simulink model "mvdc_curvvel_tracking"  (R2018b)
settings: configuration reference "Active" (kept outside this file)
undefined symbols (not defined in the file): A_VehicleReference_m2, drag_coefficient, l_front_m, l_rear_m, P_VDC_CurvDistActive, P_VDC_CurvDistEst_PT1_s, P_VDC_CurvKp, P_VDC_EmergencyBrakeAcceleration_mps2, P_VDC_EnterStandstillThreshhold_mps, P_VDC_FullControlSpeed_mps, P_VDC_FxMaxDistComp_N, P_VDC_FxMaxDistFF_N, P_VDC_FxMaxFB_N, P_VDC_FxMaxFF_N, P_VDC_FxMaxSlope_Nps, P_VDC_FxMinDistComp_N, P_VDC_FxMinDistFF_N, P_VDC_FxMinFB_N, P_VDC_FxMinFF_N, P_VDC_FxMinSlope_Nps, P_VDC_LatDeltaMaxDistComp_rad, P_VDC_LatDeltaMaxFB_rad, P_VDC_LatDeltaMaxFF_rad, P_VDC_LatDeltaMinDistComp_rad, P_VDC_LatDeltaMinFB_rad, P_VDC_LatDeltaMinFF_rad, P_VDC_LongKp, P_VDC_LowPassUSCT1, P_VDC_MaxSlopeDelta_radps, P_VDC_MinSlopeDelta_radps, P_VDC_NegativeFxStandstill_N, P_VDC_SlowControlSpeed_mps, P_VDC_UndersteerCompensationActive_b, P_VDC_UndersteerCompensationLowPassActive_b, P_VDC_UndersteerGradient, P_VDC_UseManualFF, P_VDC_VelCon_vMaxStatic_mps, P_VDC_VelDistEst_PT1_s, P_VDC_VelDistFBActive, P_VDC_VelDistFFActive, roh_air, tS, tyreradius_front_m, tyreradius_rear_m, vehiclemass_kg, WheelInertia_Front_kgm2, WheelInertia_Rear_kgm2
libraries: simulink x7, rr_general x7
settings Model: DataDictionary=mvdc_curvvel_tracking.sldd  Creator=wischnewski  LastModifiedBy=ge34qer

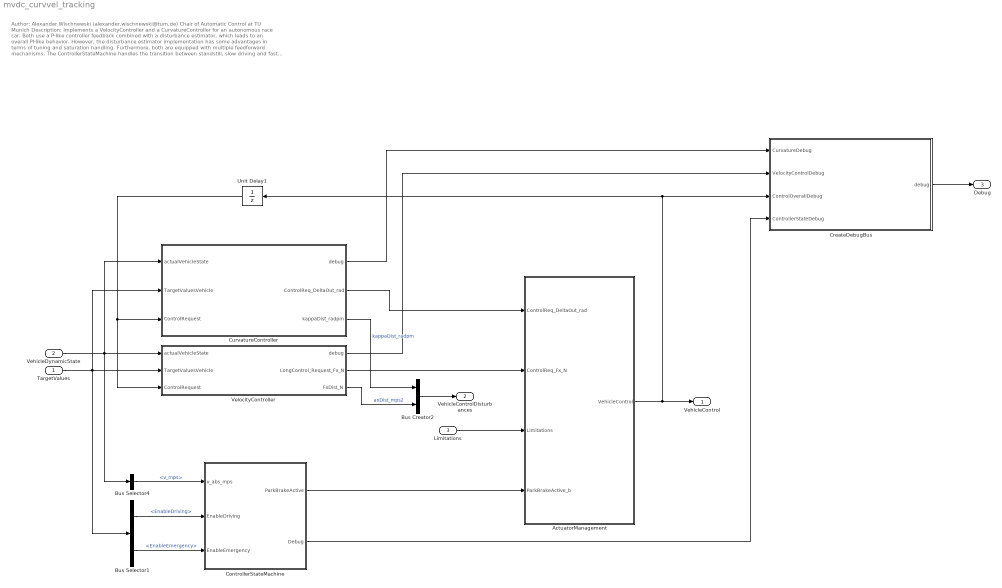
== system mvdc_curvvel_tracking ==
  note: Author: Alexander Wischnewski (alexander.wischnewski@tum.de)
      | Chair of Automatic Control at TU Munich
      |
      | Description: Implements a VelocityController and a CurvatureController for an autonomous race car. Both use a P-like controller feedback
      | combined with a disturbance estimator, which leads to an overall PI-like behavior. However, the disturbance estimator
      | implementation has some advantages in terms of tuning and saturation handling. Furthermore, both are equipped with multiple
      | feedforward mechanisms.
      |
      | The ControllerStateMachine handles the transition between standstill, slow driving and fast driving. This allows different
      | controller configurations in these scenarios.
      |
      | ActuatorManagement takes care of the final checks before the setpoints are passed to the low level actuators.
      |
      | Inputs:
      | TargetValues Setpoints and necessary feedforward information for both controllers
      | VehicleDynamicState Fused vehicle state (position, velocities, accelerations, etc.)
      | Limitations Actuator limitations
      |
      | Outputs:
      | VehicleControl Actuator setpoints used to control the vehicle
      | VehicleControlDisturbances Disturbance estimates to be used for diagnosis of vehicle status
      | Debug debug bus which includes all component debug information
  TargetValues : Inport  OutDataTypeStr=Bus: TargetValuesVehicleDynamics  PortDimensions=1  BusOutputAsStruct=on
  VehicleDynamicState : Inport  Port=2  OutDataTypeStr=Bus: VehicleDynamicState
  Limitations : Inport  Port=3  OutDataTypeStr=Bus: ActuatorLimitations  PortDimensions=1  BusOutputAsStruct=on
  ActuatorManagement : Subsystem
  Bus Creator2 : BusCreator  Inputs=2  OutDataTypeStr=Bus: VehicleControlDisturbances
      settings: InheritFromInputs=off
  Bus Selector1 : BusSelector  OutputSignals=EnableDriving,EnableEmergency
  Bus Selector4 : BusSelector  OutputSignals=v_mps
  ControllerStateMachine : Subsystem
  CreateDebugBus : Subsystem
  CurvatureController : Subsystem
  Unit Delay1 : UnitDelay  SampleTime=-1
  VelocityController : Subsystem
  VehicleControl : Outport  OutDataTypeStr=Bus: VehicleControl  BusOutputAsStruct=on
  VehicleControlDisturbances : Outport  Port=2  OutDataTypeStr=Bus: VehicleControlDisturbances  BusOutputAsStruct=on
  Debug : Outport  Port=3  OutDataTypeStr=Bus: mvdc_curvvel_tracking_debug  BusOutputAsStruct=on
  wires:
  ActuatorManagement/1(VehicleControl) -> VehicleControl/1, Unit Delay1/1, CreateDebugBus/3(ControlOverallDebug)
  VehicleDynamicState/1 -> CurvatureController/1(actualVehicleState), Bus Selector4/1, VelocityController/1(actualVehicleState)
  TargetValues/1 -> Bus Selector1/1, CurvatureController/2(TargetValuesVehicle), VelocityController/2(TargetValuesVehicle)
  Bus Selector4/1 -> ControllerStateMachine/1(v_abs_mps)  "<v_mps>"
  CurvatureController/2(ControlReq_DeltaOut_rad) -> ActuatorManagement/1(ControlReq_DeltaOut_rad)
  VelocityController/2(LongControl_Request_Fx_N) -> ActuatorManagement/2(ControlReq_Fx_N)
  Bus Creator2/1 -> VehicleControlDisturbances/1
  VelocityController/3(FxDist_N) -> Bus Creator2/2  "axDist_mps2"
  CurvatureController/3(kappaDist_radpm) -> Bus Creator2/1  "kappaDist_radpm"
  Limitations/1 -> ActuatorManagement/3(Limitations)
  Bus Selector1/1 -> ControllerStateMachine/2(EnableDriving)  "<EnableDriving>"
  Bus Selector1/2 -> ControllerStateMachine/3(EnableEmergency)  "<EnableEmergency>"
  Unit Delay1/1 -> CurvatureController/3(ControlRequest), VelocityController/3(ControlRequest)
  CurvatureController/1(debug) -> CreateDebugBus/1(CurvatureDebug)
  VelocityController/1(debug) -> CreateDebugBus/2(VelocityControlDebug)
  ControllerStateMachine/2(Debug) -> CreateDebugBus/4(ControllerStateDebug)
  CreateDebugBus/1(debug) -> Debug/1
  ControllerStateMachine/1("ParkBrakeActive ") -> ActuatorManagement/4(ParkBrakeActive_b)

== system mvdc_curvvel_tracking/ActuatorManagement ==
  ControlReq_DeltaOut_rad : Inport
  ControlReq_Fx_N : Inport  Port=2
  Limitations : Inport  Port=3
  ParkBrakeActive_b : Inport  Port=4
  Bus Creator : BusCreator  Inputs=3  OutDataTypeStr=Bus: VehicleControl
      settings: InheritFromInputs=off
  OutputChecksLong : Subsystem
  OutputChecksSteering : Subsystem
  VehicleControl : Outport  OutDataTypeStr=Bus: VehicleControl  BusOutputAsStruct=on
  wires:
  Limitations/1 -> OutputChecksLong/1(Limitations), OutputChecksSteering/1(Limitations)
  ParkBrakeActive_b/1 -> Bus Creator/3  "ParkBrakeActive"
  Bus Creator/1 -> VehicleControl/1
  ControlReq_DeltaOut_rad/1 -> OutputChecksSteering/2(delta_SteeringAngleRequest_radpm)
  OutputChecksSteering/1(RequestSteeringAngle_rad) -> Bus Creator/1  "RequestSteeringAngle_rad"
  ControlReq_Fx_N/1 -> OutputChecksLong/2(Fx_LongControlRequest_N)
  OutputChecksLong/1(RequestLongForce_N) -> Bus Creator/2  "RequestLongForce_N"

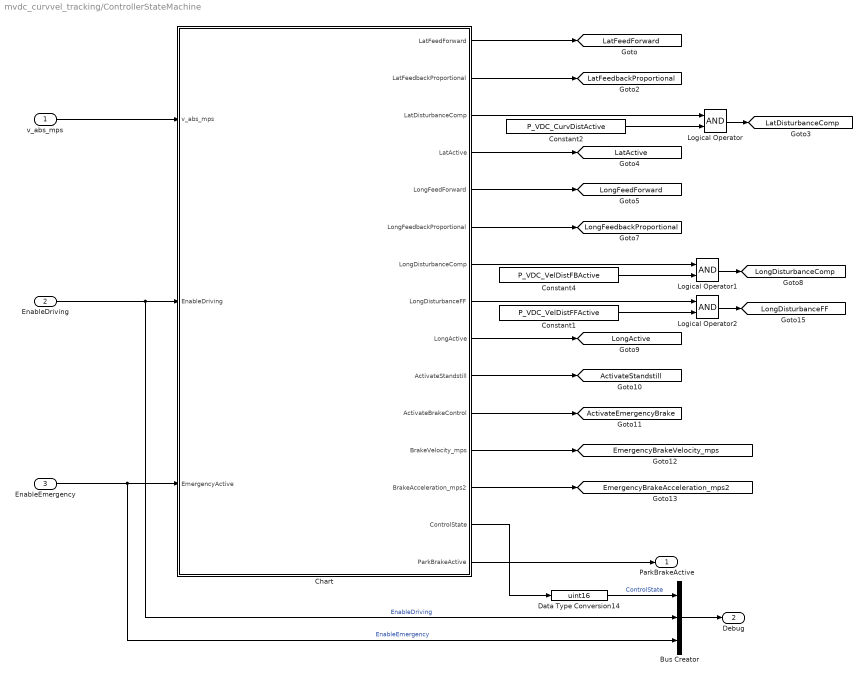
== system mvdc_curvvel_tracking/ControllerStateMachine ==
  v_abs_mps : Inport
  EnableDriving : Inport  Port=2
  EnableEmergency : Inport  Port=3
  Bus Creator : BusCreator  Inputs=3
  Chart : Stateflow chart  TreatAsAtomicUnit=on
  Constant1 : Constant  Value=P_VDC_VelDistFFActive
  Constant2 : Constant  Value=P_VDC_CurvDistActive
  Constant4 : Constant  Value=P_VDC_VelDistFBActive
  Data Type Conversion14 : DataTypeConversion  OutDataTypeStr=uint16
  Logical Operator : Logic  AllPortsSameDT=off  OutDataTypeStr=boolean
  Logical Operator1 : Logic  AllPortsSameDT=off  OutDataTypeStr=boolean
  Logical Operator2 : Logic  AllPortsSameDT=off  OutDataTypeStr=boolean
  "ParkBrakeActive " : Outport  BusOutputAsStruct=on
  Debug : Outport  Port=2
  tag scope: ActivateEmergencyBrake=global, ActivateStandstill=global, EmergencyBrakeAcceleration_mps2=global, EmergencyBrakeVelocity_mps=global, LatActive=global, LatDisturbanceComp=global, LatFeedForward=global, LatFeedbackProportional=global, LongActive=global, LongDisturbanceComp=global, LongDisturbanceFF=global, LongFeedForward=global, LongFeedbackProportional=global
  wires:
  Chart/2(LatFeedbackProportional) -> [LatFeedbackProportional]
  Chart/1(LatFeedForward) -> [LatFeedForward]
  Chart/9(LongActive) -> [LongActive]
  Logical Operator/1 -> [LatDisturbanceComp]
  Constant2/1 -> Logical Operator/2
  Constant4/1 -> Logical Operator1/2
  Logical Operator1/1 -> [LongDisturbanceComp]
  Chart/11(ActivateBrakeControl) -> [ActivateEmergencyBrake]
  Chart/13(BrakeAcceleration_mps2) -> [EmergencyBrakeAcceleration_mps2]
  Chart/12(BrakeVelocity_mps) -> [EmergencyBrakeVelocity_mps]
  Chart/10(ActivateStandstill) -> [ActivateStandstill]
  v_abs_mps/1 -> Chart/1(v_abs_mps)
  Chart/7(LongDisturbanceComp) -> Logical Operator1/1
  Chart/4(LatActive) -> [LatActive]
  Chart/5(LongFeedForward) -> [LongFeedForward]
  Chart/6(LongFeedbackProportional) -> [LongFeedbackProportional]
  Chart/3(LatDisturbanceComp) -> Logical Operator/1
  Constant1/1 -> Logical Operator2/2
  Logical Operator2/1 -> [LongDisturbanceFF]
  Chart/8(LongDisturbanceFF) -> Logical Operator2/1
  EnableDriving/1 -> Bus Creator/2, Chart/2(EnableDriving)  "EnableDriving"
  EnableEmergency/1 -> Bus Creator/3, Chart/3(EmergencyActive)  "EnableEmergency"
  Bus Creator/1 -> Debug/1
  Chart/14(ControlState) -> Data Type Conversion14/1
  Data Type Conversion14/1 -> Bus Creator/1  "ControlState"
  Chart/15(ParkBrakeActive) -> "ParkBrakeActive "/1

== system mvdc_curvvel_tracking/CreateDebugBus ==
  CurvatureDebug : Inport
  VelocityControlDebug : Inport  Port=2
  ControlOverallDebug : Inport  Port=3
  ControllerStateDebug : Inport  Port=4
  Bus Creator1 : BusCreator  Inputs=17
  Bus Selector : BusSelector  OutputSignals=Long_FB_Dist_FxReq_N,Long_FF_Dist_FxReq_N,Long_FB_VelDiff_FxReq_N,Long_FF_Traj_FxReq_N,Long_VelError_mps,Long_TargetSpeed_mps,Long_axTarget_mps2
  Bus Selector2 : BusSelector  OutputSignals=Curv_all_KappaReq_radpm,Curv_FB_Dist_DeltaReq_rad,Curv_FB_Diff_DeltaReq_rad,Curv_FF_Kappa_DeltaReq_rad,Curv_CurvError_radpm,Curv_TargetCurv_radpm
  Bus Selector3 : BusSelector  OutputSignals=ControlState,EnableDriving,EnableEmergency
  debug : Outport
  wires:
  Bus Selector/3 -> Bus Creator1/9  "<Long_FB_VelDiff_FxReq_N>"
  Bus Selector/4 -> Bus Creator1/10  "<Long_FF_Traj_FxReq_N>"
  Bus Selector/1 -> Bus Creator1/7  "<Long_FB_Dist_FxReq_N>"
  Bus Selector/5 -> Bus Creator1/11  "<Long_VelError_mps>"
  Bus Selector2/6 -> Bus Creator1/6  "<Curv_TargetCurv_radpm>"
  Bus Selector2/4 -> Bus Creator1/4  "<Curv_FF_Kappa_DeltaReq_rad>"
  Bus Selector3/2 -> Bus Creator1/16  "<EnableDriving>"
  VelocityControlDebug/1 -> Bus Selector/1
  Bus Selector2/3 -> Bus Creator1/3  "<Curv_FB_Diff_DeltaReq_rad>"
  Bus Selector3/1 -> Bus Creator1/15  "<ControlState>"
  ControllerStateDebug/1 -> Bus Selector3/1
  Bus Selector2/1 -> Bus Creator1/1  "<Curv_all_KappaReq_radpm>"
  Bus Selector2/5 -> Bus Creator1/5  "<Curv_CurvError_radpm>"
  Bus Selector3/3 -> Bus Creator1/17  "<EnableEmergency>"
  Bus Selector2/2 -> Bus Creator1/2  "<Curv_FB_Dist_DeltaReq_rad>"
  Bus Creator1/1 -> debug/1
  ControlOverallDebug/1 -> Bus Creator1/14  "CO"
  Bus Selector/7 -> Bus Creator1/13  "<Long_axTarget_mps2>"
  Bus Selector/2 -> Bus Creator1/8  "<Long_FF_Dist_FxReq_N>"
  CurvatureDebug/1 -> Bus Selector2/1
  Bus Selector/6 -> Bus Creator1/12  "<Long_TargetSpeed_mps>"

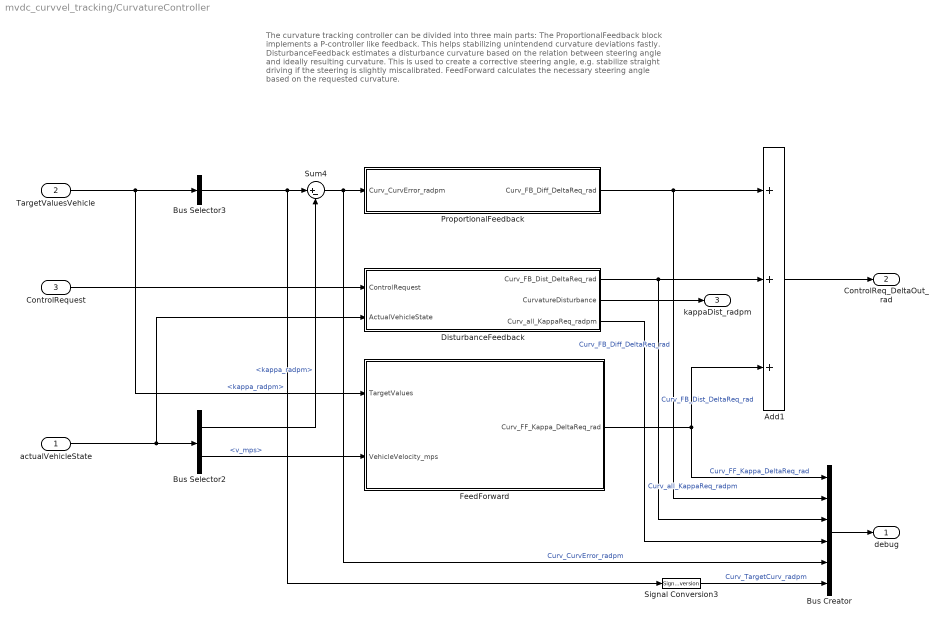
== system mvdc_curvvel_tracking/CurvatureController ==
  note: The curvature tracking controller can be divided into three main parts:
      |
      | The ProportionalFeedback block implements a P-controller like feedback. This helps stabilizing unintendend curvature deviations fastly.
      |
      | DisturbanceFeedback estimates a disturbance curvature based on the relation between steering angle and ideally resulting curvature. This is
      | used to create a corrective steering angle, e.g. stabilize straight driving if the steering is slightly miscalibrated.
      |
      | FeedForward calculates the necessary steering angle based on the requested curvature.
  actualVehicleState : Inport
  TargetValuesVehicle : Inport  Port=2
  ControlRequest : Inport  Port=3
  Add1 : Sum  Inputs=+++
  Bus Creator : BusCreator  Inputs=6
  Bus Selector2 : BusSelector  OutputSignals=kappa_radpm,v_mps
  Bus Selector3 : BusSelector  OutputSignals=kappa_radpm
  DisturbanceFeedback : Subsystem
  FeedForward : Subsystem
  ProportionalFeedback : Subsystem
  Signal Conversion3 : SignalConversion  OverrideOpt=off
  Sum4 : Sum  Inputs=|+-
  debug : Outport
  ControlReq_DeltaOut_rad : Outport  Port=2
  kappaDist_radpm : Outport  Port=3
  wires:
  Bus Selector2/1 -> Sum4/2  "<kappa_radpm>"
  Sum4/1 -> Bus Creator/5, ProportionalFeedback/1(Curv_CurvError_radpm)  "Curv_CurvError_radpm"
  Bus Selector2/2 -> FeedForward/2(VehicleVelocity_mps)  "<v_mps>"
  actualVehicleState/1 -> DisturbanceFeedback/2(ActualVehicleState), Bus Selector2/1
  TargetValuesVehicle/1 -> FeedForward/1(TargetValues), Bus Selector3/1
  Signal Conversion3/1 -> Bus Creator/6  "Curv_TargetCurv_radpm"
  Bus Creator/1 -> debug/1
  Bus Selector3/1 -> Sum4/1, Signal Conversion3/1  "<kappa_radpm>"
  Add1/1 -> ControlReq_DeltaOut_rad/1
  ProportionalFeedback/1(Curv_FB_Diff_DeltaReq_rad) -> Add1/1, Bus Creator/2  "Curv_FB_Diff_DeltaReq_rad"
  DisturbanceFeedback/1(Curv_FB_Dist_DeltaReq_rad) -> Add1/2, Bus Creator/3  "Curv_FB_Dist_DeltaReq_rad"
  FeedForward/1(Curv_FF_Kappa_DeltaReq_rad) -> Bus Creator/1, Add1/3  "Curv_FF_Kappa_DeltaReq_rad"
  ControlRequest/1 -> DisturbanceFeedback/1(ControlRequest)
  DisturbanceFeedback/2(CurvatureDisturbance) -> kappaDist_radpm/1
  DisturbanceFeedback/3(Curv_all_KappaReq_radpm) -> Bus Creator/4  "Curv_all_KappaReq_radpm"

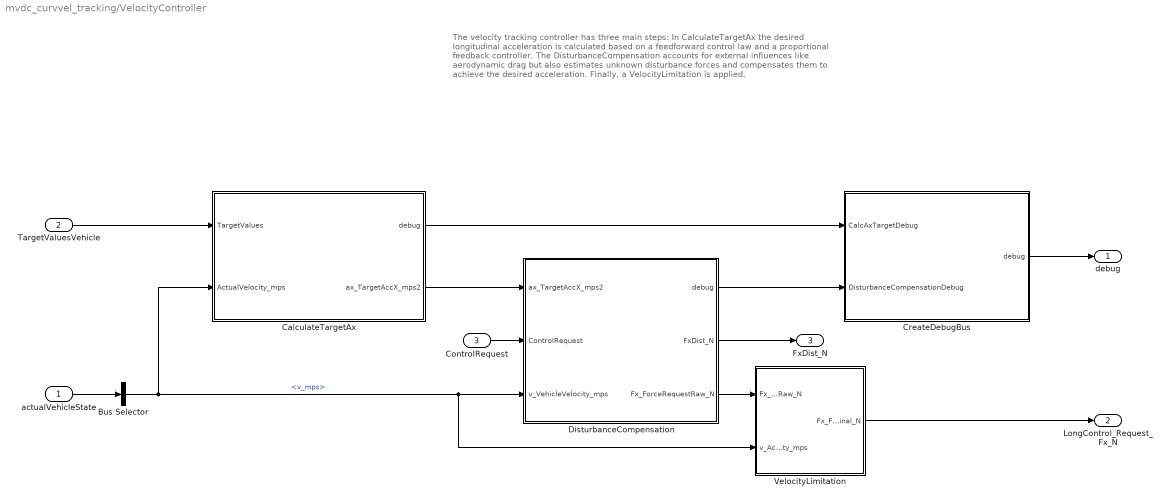
== system mvdc_curvvel_tracking/VelocityController ==
  note: The velocity tracking controller has three main steps:
      |
      | In CalculateTargetAx the desired longitudinal acceleration is calculated based on a
      | feedforward control law and a proportional feedback controller.
      |
      | The DisturbanceCompensation accounts for external influences like aerodynamic drag
      | but also estimates unknown disturbance forces and compensates them to achieve
      | the desired acceleration.
      |
      | Finally, a VelocityLimitation is applied.
  actualVehicleState : Inport
  TargetValuesVehicle : Inport  Port=2
  ControlRequest : Inport  Port=3
  Bus Selector : BusSelector  OutputSignals=v_mps
  CalculateTargetAx : Subsystem
  CreateDebugBus : Subsystem
  DisturbanceCompensation : Subsystem
  VelocityLimitation : Subsystem
  debug : Outport
  LongControl_Request_Fx_N : Outport  Port=2
  FxDist_N : Outport  Port=3
  wires:
  Bus Selector/1 -> VelocityLimitation/2(v_ActualVelocity_mps), DisturbanceCompensation/3(v_VehicleVelocity_mps), CalculateTargetAx/2(ActualVelocity_mps)  "<v_mps>"
  TargetValuesVehicle/1 -> CalculateTargetAx/1(TargetValues)
  actualVehicleState/1 -> Bus Selector/1
  DisturbanceCompensation/2(FxDist_N) -> FxDist_N/1
  VelocityLimitation/1(Fx_ForceRequestFinal_N) -> LongControl_Request_Fx_N/1
  CalculateTargetAx/2(ax_TargetAccX_mps2) -> DisturbanceCompensation/1(ax_TargetAccX_mps2)
  ControlRequest/1 -> DisturbanceCompensation/2(ControlRequest)
  DisturbanceCompensation/3(Fx_ForceRequestRaw_N) -> VelocityLimitation/1(Fx_ForceRequestRaw_N)
  CalculateTargetAx/1(debug) -> CreateDebugBus/1(CalcAxTargetDebug)
  DisturbanceCompensation/1(debug) -> CreateDebugBus/2(DisturbanceCompensationDebug)
  CreateDebugBus/1(debug) -> debug/1

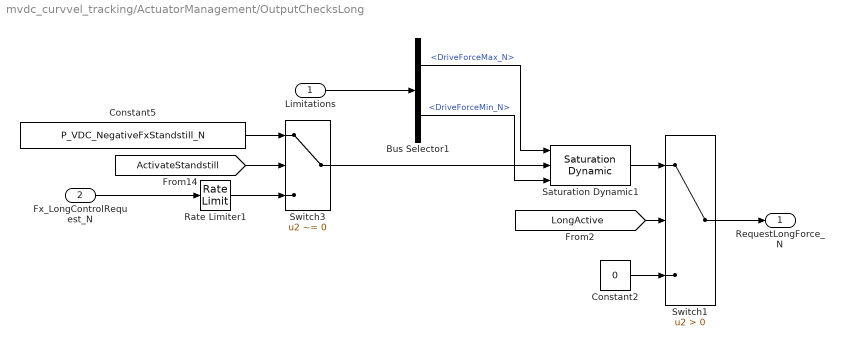
== system mvdc_curvvel_tracking/ActuatorManagement/OutputChecksLong ==
  Limitations : Inport
  Fx_LongControlRequest_N : Inport  Port=2
  Bus Selector1 : BusSelector  OutputSignals=DriveForceMax_N,DriveForceMin_N
  Constant2 : Constant  Value=0
  Constant5 : Constant  Value=P_VDC_NegativeFxStandstill_N
  Rate Limiter1 : RateLimiter  RisingSlewLimit=P_VDC_FxMaxSlope_Nps  FallingSlewLimit=P_VDC_FxMinSlope_Nps  SampleTimeMode=inherited
  Saturation Dynamic1 : simulink/Discontinuities/Saturation Dynamic  OutMin=[]  OutMax=[]  OutDataTypeStr=Inherit: Same as second input  OutDataType=fixdt(1, 16)  OutScaling=2^-10  DoSatur=off
  Switch1 : Switch  Criteria=u2 > Threshold
  Switch3 : Switch  Criteria=u2 ~= 0
  RequestLongForce_N : Outport
  wires:
  Saturation Dynamic1/1 -> Switch1/1
  Rate Limiter1/1 -> Switch3/3
  Bus Selector1/1 -> Saturation Dynamic1/1  "<DriveForceMax_N>"
  [ActivateStandstill] -> Switch3/2
  Constant2/1 -> Switch1/3
  Bus Selector1/2 -> Saturation Dynamic1/3  "<DriveForceMin_N>"
  Switch3/1 -> Saturation Dynamic1/2
  Constant5/1 -> Switch3/1
  [LongActive] -> Switch1/2
  Switch1/1 -> RequestLongForce_N/1
  Fx_LongControlRequest_N/1 -> Rate Limiter1/1
  Limitations/1 -> Bus Selector1/1

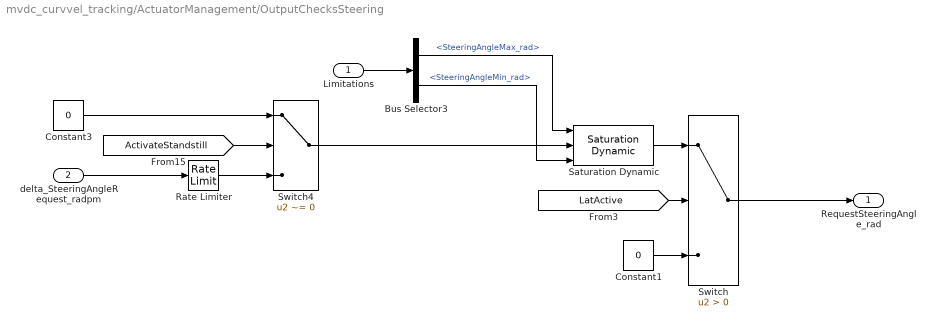
== system mvdc_curvvel_tracking/ActuatorManagement/OutputChecksSteering ==
  Limitations : Inport
  delta_SteeringAngleRequest_radpm : Inport  Port=2
  Bus Selector3 : BusSelector  OutputSignals=SteeringAngleMax_rad,SteeringAngleMin_rad
  Constant1 : Constant  Value=0
  Constant3 : Constant  Value=0
  Rate Limiter : RateLimiter  RisingSlewLimit=P_VDC_MaxSlopeDelta_radps  FallingSlewLimit=P_VDC_MinSlopeDelta_radps  SampleTimeMode=inherited
  Saturation Dynamic : simulink/Discontinuities/Saturation Dynamic  OutMin=[]  OutMax=[]  OutDataTypeStr=Inherit: Same as second input  OutDataType=fixdt(1, 16)  OutScaling=2^-10  DoSatur=off
  Switch : Switch  Criteria=u2 > Threshold
  Switch4 : Switch  Criteria=u2 ~= 0
  RequestSteeringAngle_rad : Outport
  wires:
  Switch4/1 -> Saturation Dynamic/2
  Constant3/1 -> Switch4/1
  Saturation Dynamic/1 -> Switch/1
  [ActivateStandstill] -> Switch4/2
  Rate Limiter/1 -> Switch4/3
  Bus Selector3/1 -> Saturation Dynamic/1  "<SteeringAngleMax_rad>"
  Bus Selector3/2 -> Saturation Dynamic/3  "<SteeringAngleMin_rad>"
  Constant1/1 -> Switch/3
  [LatActive] -> Switch/2
  delta_SteeringAngleRequest_radpm/1 -> Rate Limiter/1
  Switch/1 -> RequestSteeringAngle_rad/1
  Limitations/1 -> Bus Selector3/1

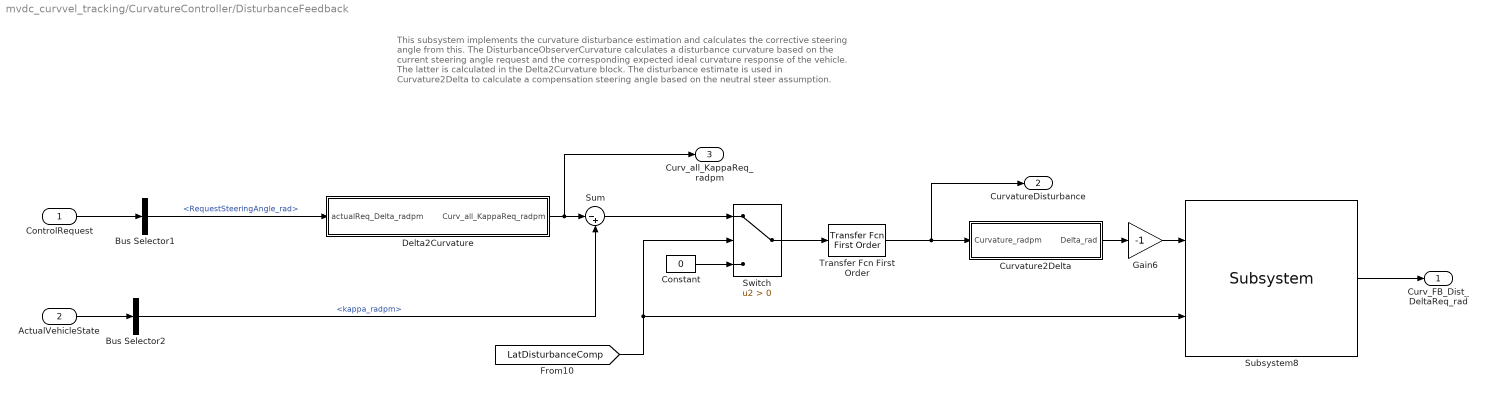
== system mvdc_curvvel_tracking/CurvatureController/DisturbanceFeedback ==
  note: This subsystem implements the curvature disturbance estimation and calculates the corrective steering angle from this.
      |
      | The DisturbanceObserverCurvature calculates a disturbance curvature based on the current steering angle request
      | and the corresponding expected ideal curvature response of the vehicle. The latter is calculated in the Delta2Curvature block.
      | The disturbance estimate is used in Curvature2Delta to calculate a compensation steering angle based on the neutral
      | steer assumption.
  ControlRequest : Inport
  ActualVehicleState : Inport  Port=2
  Bus Selector1 : BusSelector  OutputSignals=RequestSteeringAngle_rad
  Bus Selector2 : BusSelector  OutputSignals=kappa_radpm
  Constant : Constant  Value=0
  Curvature2Delta : Subsystem
  Delta2Curvature : Subsystem
  Gain6 : Gain  Gain=-1
  Subsystem8 : rr_general/Subsystem  UpperLimit=P_VDC_LatDeltaMaxDistComp_rad  LowerLimit=P_VDC_LatDeltaMinDistComp_rad
  Sum : Sum  Inputs=|-+
  Switch : Switch  Criteria=u2 > Threshold
  Transfer Fcn First Order : simulink/Discrete/Transfer Fcn First Order  PoleZ=exp(-tS/P_VDC_CurvDistEst_PT1_s)  ICPrevOutput=0.0  DoSatur=off
      settings: SourceProductName=Simulink
  Curv_FB_Dist_DeltaReq_rad : Outport
  CurvatureDisturbance : Outport  Port=2
  Curv_all_KappaReq_radpm : Outport  Port=3
  wires:
  Gain6/1 -> Subsystem8/1
  [LatDisturbanceComp] -> Subsystem8/2, Switch/2
  Curvature2Delta/1(Delta_rad) -> Gain6/1
  Subsystem8/1 -> Curv_FB_Dist_DeltaReq_rad/1
  ControlRequest/1 -> Bus Selector1/1
  Delta2Curvature/1(Curv_all_KappaReq_radpm) -> Curv_all_KappaReq_radpm/1, Sum/1
  Transfer Fcn First Order/1 -> CurvatureDisturbance/1, Curvature2Delta/1(Curvature_radpm)
  ActualVehicleState/1 -> Bus Selector2/1
  Bus Selector2/1 -> Sum/2  "<kappa_radpm>"
  Sum/1 -> Switch/1
  Constant/1 -> Switch/3
  Switch/1 -> Transfer Fcn First Order/1
  Bus Selector1/1 -> Delta2Curvature/1(actualReq_Delta_radpm)  "<RequestSteeringAngle_rad>"

== system mvdc_curvvel_tracking/CurvatureController/FeedForward ==
  note: Two options are available for feedforward generation:
      |
      | The top option uses a direct feed-through of a externally
      | supplied steering angle.
      |
      | The bottom option calculates the steering feedforward based on the
      | curvature setpoint and an additional feedforward curvature value kappaFF_radpm.
  TargetValues : Inport
  VehicleVelocity_mps : Inport  Port=2
  Bus Selector : BusSelector  OutputSignals=ManualFF_Delta_rad,kappa_radpm,kappaFF_radpm
  Constant2 : Constant  Value=P_VDC_UseManualFF
  Curvature2Delta : Subsystem
  Subsystem7 : rr_general/Subsystem  UpperLimit=P_VDC_LatDeltaMaxFF_rad  LowerLimit=P_VDC_LatDeltaMinFF_rad
  Sum : Sum  Inputs=++|
  Switch3 : Switch  Criteria=u2 ~= 0
  Curv_FF_Kappa_DeltaReq_rad : Outport
  wires:
  [LatFeedForward] -> Subsystem7/2
  Constant2/1 -> Switch3/2
  Sum/1 -> Curvature2Delta/1(TargetCurvature_radpm)
  Switch3/1 -> Subsystem7/1
  Curvature2Delta/1(SteeringAngle_rad) -> Switch3/3
  Subsystem7/1 -> Curv_FF_Kappa_DeltaReq_rad/1
  TargetValues/1 -> Bus Selector/1
  Bus Selector/1 -> Switch3/1  "<ManualFF_Delta_rad>"
  VehicleVelocity_mps/1 -> Curvature2Delta/2(ActualVelocity_mps)
  Bus Selector/3 -> Sum/2  "<kappaFF_radpm>"
  Bus Selector/2 -> Sum/1  "<kappa_radpm>"

== system mvdc_curvvel_tracking/CurvatureController/ProportionalFeedback ==
  Curv_CurvError_radpm : Inport
  Gain3 : Gain  Gain=P_VDC_CurvKp
  Subsystem9 : rr_general/Subsystem  UpperLimit=P_VDC_LatDeltaMaxFB_rad  LowerLimit=P_VDC_LatDeltaMinFB_rad
  Curv_FB_Diff_DeltaReq_rad : Outport
  wires:
  [LatFeedbackProportional] -> Subsystem9/2
  Subsystem9/1 -> Curv_FB_Diff_DeltaReq_rad/1
  Curv_CurvError_radpm/1 -> Gain3/1
  Gain3/1 -> Subsystem9/1

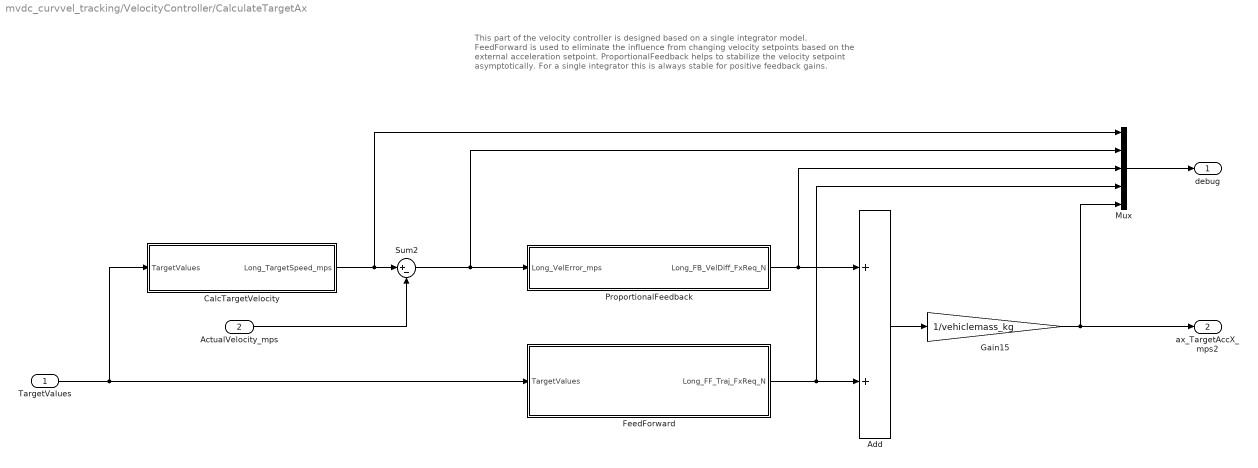
== system mvdc_curvvel_tracking/VelocityController/CalculateTargetAx ==
  note: This part of the velocity controller is designed based on a single integrator model.
      |
      | FeedForward is used to eliminate the influence from changing velocity setpoints based
      | on the external acceleration setpoint.
      |
      | ProportionalFeedback helps to stabilize the velocity setpoint asymptotically. For a single
      | integrator this is always stable for positive feedback gains.
  TargetValues : Inport
  ActualVelocity_mps : Inport  Port=2
  Add : Sum
  CalcTargetVelocity : Subsystem
  FeedForward : Subsystem
  Gain15 : Gain  Gain=1/vehiclemass_kg
  Mux : Mux  Inputs=5
  ProportionalFeedback : Subsystem
  Sum2 : Sum  Inputs=|+-
  debug : Outport
  ax_TargetAccX_mps2 : Outport  Port=2
  wires:
  TargetValues/1 -> CalcTargetVelocity/1(TargetValues), FeedForward/1(TargetValues)
  ProportionalFeedback/1(Long_FB_VelDiff_FxReq_N) -> Mux/3, Add/1
  FeedForward/1(Long_FF_Traj_FxReq_N) -> Mux/4, Add/2
  Add/1 -> Gain15/1
  Gain15/1 -> Mux/5, ax_TargetAccX_mps2/1
  Mux/1 -> debug/1
  CalcTargetVelocity/1(Long_TargetSpeed_mps) -> Mux/1, Sum2/1
  ActualVelocity_mps/1 -> Sum2/2
  Sum2/1 -> Mux/2, ProportionalFeedback/1(Long_VelError_mps)

== system mvdc_curvvel_tracking/VelocityController/CreateDebugBus ==
  CalcAxTargetDebug : Inport
  DisturbanceCompensationDebug : Inport  Port=2
  Bus Creator : BusCreator  Inputs=7
  Demux : Demux  Outputs=5
  Demux1 : Demux  Outputs=2
  debug : Outport
  wires:
  CalcAxTargetDebug/1 -> Demux/1
  Bus Creator/1 -> debug/1
  Demux/3 -> Bus Creator/3  "Long_FB_VelDiff_FxReq_N"
  Demux1/1 -> Bus Creator/6  "Long_FB_Dist_FxReq_N"
  Demux/1 -> Bus Creator/1  "Long_TargetSpeed_mps"
  Demux/2 -> Bus Creator/2  "Long_VelError_mps"
  Demux/4 -> Bus Creator/4  "Long_FF_Traj_FxReq_N"
  Demux/5 -> Bus Creator/5  "Long_axTarget_mps2"
  Demux1/2 -> Bus Creator/7  "Long_FF_Dist_FxReq_N"
  DisturbanceCompensationDebug/1 -> Demux1/1

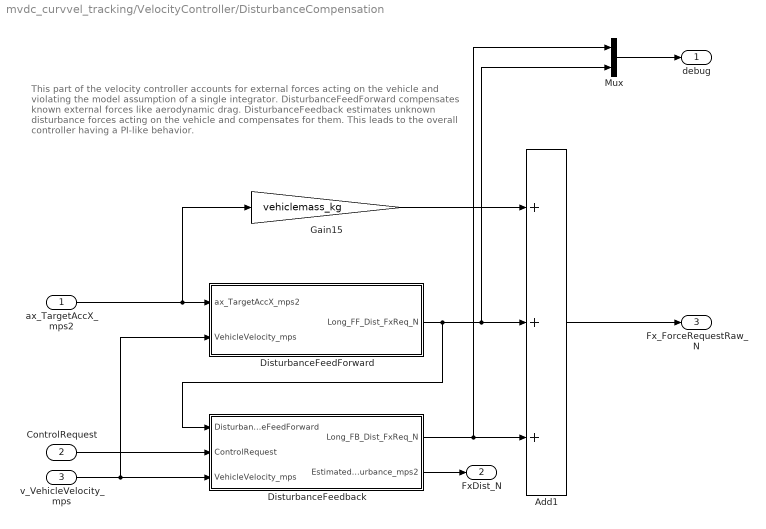
== system mvdc_curvvel_tracking/VelocityController/DisturbanceCompensation ==
  note: This part of the velocity controller accounts for external forces acting on the vehicle and
      | violating the model assumption of a single integrator.
      |
      | DisturbanceFeedForward compensates known external forces like aerodynamic drag.
      |
      | DisturbanceFeedback estimates unknown disturbance forces acting on the vehicle
      | and compensates for them. This leads to the overall controller having a PI-like behavior.
  ax_TargetAccX_mps2 : Inport
  ControlRequest : Inport  Port=2
  v_VehicleVelocity_mps : Inport  Port=3
  Add1 : Sum  Inputs=+++
  DisturbanceFeedForward : Subsystem
  DisturbanceFeedback : Subsystem
  Gain15 : Gain  Gain=vehiclemass_kg
  Mux : Mux  Inputs=2
  debug : Outport
  FxDist_N : Outport  Port=2
  Fx_ForceRequestRaw_N : Outport  Port=3
  wires:
  v_VehicleVelocity_mps/1 -> DisturbanceFeedForward/2(VehicleVelocity_mps), DisturbanceFeedback/3(VehicleVelocity_mps)
  DisturbanceFeedForward/1(Long_FF_Dist_FxReq_N) -> DisturbanceFeedback/1(DisturbanceFeedForward), Mux/2, Add1/2
  ControlRequest/1 -> DisturbanceFeedback/2(ControlRequest)
  Add1/1 -> Fx_ForceRequestRaw_N/1
  DisturbanceFeedback/1(Long_FB_Dist_FxReq_N) -> Mux/1, Add1/3
  ax_TargetAccX_mps2/1 -> Gain15/1, DisturbanceFeedForward/1(ax_TargetAccX_mps2)
  Gain15/1 -> Add1/1
  Mux/1 -> debug/1
  DisturbanceFeedback/2(EstimatedAccXDisturbance_mps2) -> FxDist_N/1

== system mvdc_curvvel_tracking/VelocityController/VelocityLimitation ==
  note: This subsystem implements a velocity limitation. If the vehicle reaches the velocity limit,
      | positive forces are no longer passed to the actuators.
  Fx_ForceRequestRaw_N : Inport
  v_ActualVelocity_mps : Inport  Port=2
  Compare To Zero : simulink/Logic and Bit Operations/Compare To Zero  relop=>=  OutDataTypeStr=boolean
  Constant1 : Constant  Value=P_VDC_VelCon_vMaxStatic_mps
  Saturation : Saturate  UpperLimit=0  LowerLimit=-inf
  Sum3 : Sum  Inputs=-+|
  Switch1 : Switch  Criteria=u2 > Threshold
  Fx_ForceRequestFinal_N : Outport
  wires:
  Fx_ForceRequestRaw_N/1 -> Switch1/3, Saturation/1
  Compare To Zero/1 -> Switch1/2
  Saturation/1 -> Switch1/1
  Switch1/1 -> Fx_ForceRequestFinal_N/1
  Sum3/1 -> Compare To Zero/1
  v_ActualVelocity_mps/1 -> Sum3/2
  Constant1/1 -> Sum3/1

== system mvdc_curvvel_tracking/CurvatureController/DisturbanceFeedback/Curvature2Delta ==
  Curvature_radpm : Inport
  Gain4 : Gain  Gain=l_front_m+l_rear_m
  Delta_rad : Outport
  wires:
  Gain4/1 -> Delta_rad/1
  Curvature_radpm/1 -> Gain4/1

== system mvdc_curvvel_tracking/CurvatureController/DisturbanceFeedback/Delta2Curvature ==
  actualReq_Delta_radpm : Inport
  Gain2 : Gain  Gain=1/(l_front_m+l_rear_m)
  Curv_all_KappaReq_radpm : Outport
  wires:
  Gain2/1 -> Curv_all_KappaReq_radpm/1
  actualReq_Delta_radpm/1 -> Gain2/1

== system mvdc_curvvel_tracking/CurvatureController/FeedForward/Curvature2Delta ==
  note: This subsystem uses an inverse linear steady state model to calculate the steering angle from the target
      | curvature. As an additional option it is possible to enable an understeer compensation based
      | on the linear single track model.
  TargetCurvature_radpm : Inport
  ActualVelocity_mps : Inport  Port=2
  InverseSteadyStateLinearModel : Subsystem
  SteeringAngle_rad : Outport
  wires:
  TargetCurvature_radpm/1 -> InverseSteadyStateLinearModel/2(CurvatureRequest)
  InverseSteadyStateLinearModel/1(SteeringAngle_rad) -> SteeringAngle_rad/1
  ActualVelocity_mps/1 -> InverseSteadyStateLinearModel/1(VehicleVelocity_mps)

== system mvdc_curvvel_tracking/VelocityController/CalculateTargetAx/CalcTargetVelocity ==
  TargetValues : Inport
  Bus Selector1 : BusSelector  OutputSignals=v_mps
  Saturation : Saturate  UpperLimit=P_VDC_VelCon_vMaxStatic_mps  LowerLimit=0
  Switch5 : Switch  Criteria=u2 ~= 0
  Long_TargetSpeed_mps : Outport
  wires:
  [EmergencyBrakeVelocity_mps] -> Switch5/1
  [ActivateEmergencyBrake] -> Switch5/2
  Saturation/1 -> Long_TargetSpeed_mps/1
  Switch5/1 -> Saturation/1
  Bus Selector1/1 -> Switch5/3  "<v_mps>"
  TargetValues/1 -> Bus Selector1/1

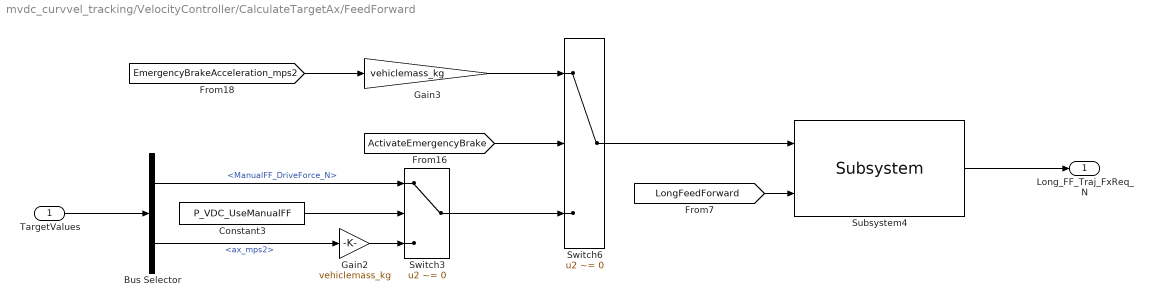
== system mvdc_curvvel_tracking/VelocityController/CalculateTargetAx/FeedForward ==
  TargetValues : Inport
  Bus Selector : BusSelector  OutputSignals=ManualFF_DriveForce_N,ax_mps2
  Constant3 : Constant  Value=P_VDC_UseManualFF
  Gain2 : Gain  Gain=vehiclemass_kg
  Gain3 : Gain  Gain=vehiclemass_kg
  Subsystem4 : rr_general/Subsystem  UpperLimit=P_VDC_FxMaxFF_N  LowerLimit=P_VDC_FxMinFF_N
  Switch3 : Switch  Criteria=u2 ~= 0
  Switch6 : Switch  Criteria=u2 ~= 0
  Long_FF_Traj_FxReq_N : Outport
  wires:
  Switch6/1 -> Subsystem4/1
  Constant3/1 -> Switch3/2
  Switch3/1 -> Switch6/3
  Gain3/1 -> Switch6/1
  Bus Selector/1 -> Switch3/1  "<ManualFF_DriveForce_N>"
  [EmergencyBrakeAcceleration_mps2] -> Gain3/1
  [LongFeedForward] -> Subsystem4/2
  Gain2/1 -> Switch3/3
  Bus Selector/2 -> Gain2/1  "<ax_mps2>"
  Subsystem4/1 -> Long_FF_Traj_FxReq_N/1
  TargetValues/1 -> Bus Selector/1
  [ActivateEmergencyBrake] -> Switch6/2

== system mvdc_curvvel_tracking/VelocityController/CalculateTargetAx/ProportionalFeedback ==
  Long_VelError_mps : Inport
  Gain1 : Gain  Gain=P_VDC_LongKp
  Subsystem3 : rr_general/Subsystem  UpperLimit=P_VDC_FxMaxFB_N  LowerLimit=P_VDC_FxMinFB_N
  Long_FB_VelDiff_FxReq_N : Outport
  wires:
  Gain1/1 -> Subsystem3/1
  [LongFeedbackProportional] -> Subsystem3/2
  Subsystem3/1 -> Long_FB_VelDiff_FxReq_N/1
  Long_VelError_mps/1 -> Gain1/1

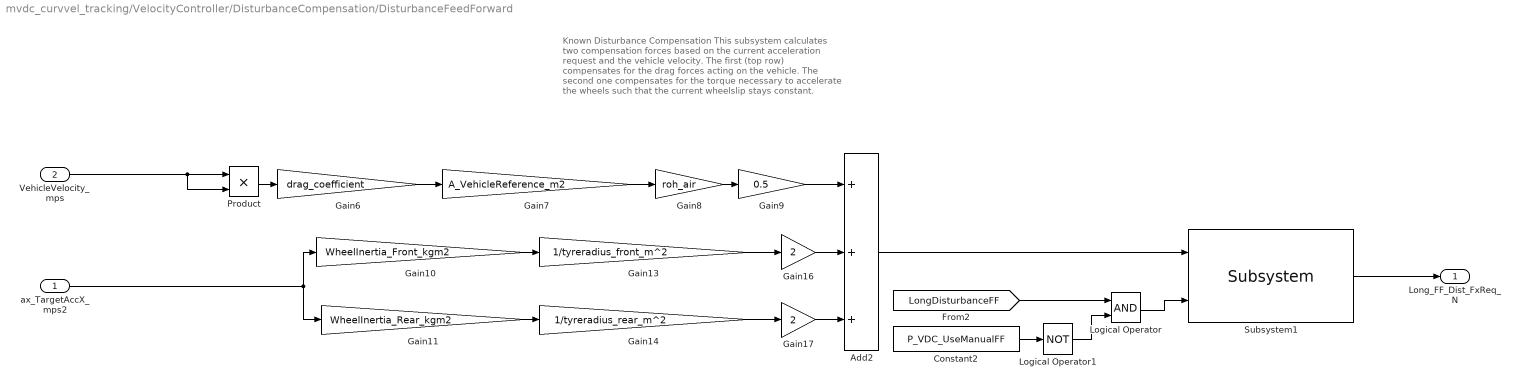
== system mvdc_curvvel_tracking/VelocityController/DisturbanceCompensation/DisturbanceFeedForward ==
  note: Known Disturbance Compensation
      |
      | This subsystem calculates two compensation forces based
      | on the current acceleration request and the vehicle velocity.
      | The first (top row) compensates for the drag forces acting
      | on the vehicle. The second one compensates for the
      | torque necessary to accelerate the wheels such that the
      | current wheelslip stays constant.
  ax_TargetAccX_mps2 : Inport
  VehicleVelocity_mps : Inport  Port=2
  Add2 : Sum  Inputs=+++
  Constant2 : Constant  Value=P_VDC_UseManualFF
  Gain10 : Gain  Gain=WheelInertia_Front_kgm2
  Gain11 : Gain  Gain=WheelInertia_Rear_kgm2
  Gain13 : Gain  Gain=1/tyreradius_front_m^2
  Gain14 : Gain  Gain=1/tyreradius_rear_m^2
  Gain16 : Gain  Gain=2
  Gain17 : Gain  Gain=2
  Gain6 : Gain  Gain=drag_coefficient
  Gain7 : Gain  Gain=A_VehicleReference_m2
  Gain8 : Gain  Gain=roh_air
  Gain9 : Gain  Gain=0.5
  Logical Operator : Logic  AllPortsSameDT=off  OutDataTypeStr=boolean
  Logical Operator1 : Logic  Operator=NOT  Inputs=1  AllPortsSameDT=off  OutDataTypeStr=boolean
  Product : Product
  Subsystem1 : rr_general/Subsystem  UpperLimit=P_VDC_FxMaxDistFF_N  LowerLimit=P_VDC_FxMinDistFF_N
  Long_FF_Dist_FxReq_N : Outport
  wires:
  Gain11/1 -> Gain14/1
  Add2/1 -> Subsystem1/1
  ax_TargetAccX_mps2/1 -> Gain11/1, Gain10/1
  Gain14/1 -> Gain17/1
  Gain16/1 -> Add2/2
  Gain17/1 -> Add2/3
  Gain13/1 -> Gain16/1
  Gain8/1 -> Gain9/1
  Product/1 -> Gain6/1
  VehicleVelocity_mps/1 -> Product/2, Product/1
  Gain10/1 -> Gain13/1
  Gain7/1 -> Gain8/1
  Gain6/1 -> Gain7/1
  Gain9/1 -> Add2/1
  Subsystem1/1 -> Long_FF_Dist_FxReq_N/1
  [LongDisturbanceFF] -> Logical Operator/1
  Logical Operator/1 -> Subsystem1/2
  Constant2/1 -> Logical Operator1/1
  Logical Operator1/1 -> Logical Operator/2

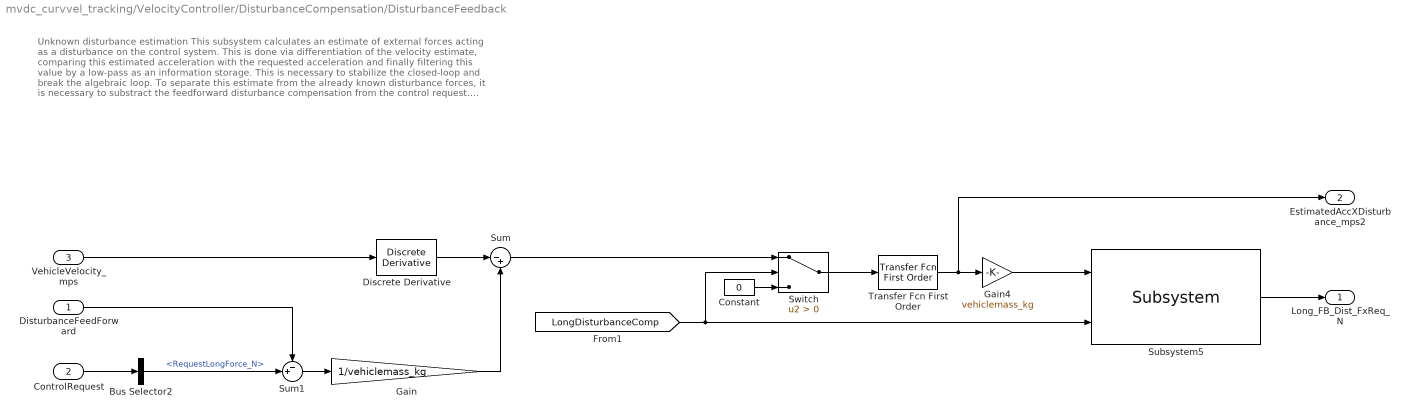
== system mvdc_curvvel_tracking/VelocityController/DisturbanceCompensation/DisturbanceFeedback ==
  note: Unknown disturbance estimation
      |
      | This subsystem calculates an estimate of external forces acting as a disturbance on the
      | control system. This is done via differentiation of the velocity estimate, comparing this
      | estimated acceleration with the requested acceleration and finally filtering this value
      | by a low-pass as an information storage. This is necessary to stabilize the closed-loop and
      | break the algebraic loop.
      |
      | To separate this estimate from the already known disturbance forces,
      | it is necessary to substract the feedforward disturbance compensation from the
      | control request. The disturbance observer therefore doesnt notice these forces are there.
  DisturbanceFeedForward : Inport
  ControlRequest : Inport  Port=2
  VehicleVelocity_mps : Inport  Port=3
  Bus Selector2 : BusSelector  OutputSignals=RequestLongForce_N
  Constant : Constant  Value=0
  Discrete Derivative : simulink/Discrete/Discrete Derivative  gainval=1.0  ICPrevScaledInput=0.0  OutMin=[]  OutMax=[]  OutDataType=fixdt(1, 16)  OutScaling=2^-10  DoSatur=off
  Gain : Gain  Gain=1/vehiclemass_kg
  Gain4 : Gain  Gain=vehiclemass_kg
  Subsystem5 : rr_general/Subsystem  UpperLimit=P_VDC_FxMaxDistComp_N  LowerLimit=P_VDC_FxMinDistComp_N
  Sum : Sum  Inputs=|-+
  Sum1 : Sum  Inputs=-+|
  Switch : Switch  Criteria=u2 > Threshold
  Transfer Fcn First Order : simulink/Discrete/Transfer Fcn First Order  PoleZ=exp(-tS/P_VDC_VelDistEst_PT1_s)  ICPrevOutput=0.0  DoSatur=off
      settings: SourceProductName=Simulink
  Long_FB_Dist_FxReq_N : Outport
  EstimatedAccXDisturbance_mps2 : Outport  Port=2
  wires:
  Gain4/1 -> Subsystem5/1
  Subsystem5/1 -> Long_FB_Dist_FxReq_N/1
  Transfer Fcn First Order/1 -> Gain4/1, EstimatedAccXDisturbance_mps2/1
  Sum1/1 -> Gain/1
  Bus Selector2/1 -> Sum1/2  "<RequestLongForce_N>"
  ControlRequest/1 -> Bus Selector2/1
  VehicleVelocity_mps/1 -> Discrete Derivative/1
  DisturbanceFeedForward/1 -> Sum1/1
  Discrete Derivative/1 -> Sum/1
  Gain/1 -> Sum/2
  Switch/1 -> Transfer Fcn First Order/1
  Sum/1 -> Switch/1
  [LongDisturbanceComp] -> Subsystem5/2, Switch/2
  Constant/1 -> Switch/3

== system mvdc_curvvel_tracking/CurvatureController/FeedForward/Curvature2Delta/InverseSteadyStateLinearModel ==
  VehicleVelocity_mps : Inport
  CurvatureRequest : Inport  Port=2
  Constant3 : Constant  Value=P_VDC_UndersteerCompensationActive_b
  NeutralSteer : Subsystem
  Switch1 : Switch  Criteria=u2 > Threshold
  USCompensation_LinearModel : Subsystem
  SteeringAngle_rad : Outport
  wires:
  Constant3/1 -> Switch1/2
  NeutralSteer/1(SteeringAngle_rad) -> Switch1/3
  CurvatureRequest/1 -> USCompensation_LinearModel/2(CurvatureRequest_radpm), NeutralSteer/1(CurvatureRequest_radpm)
  USCompensation_LinearModel/1(USComp_SteeringAngle_rad) -> Switch1/1
  VehicleVelocity_mps/1 -> USCompensation_LinearModel/1(VehicleVelocity_mps)
  Switch1/1 -> SteeringAngle_rad/1

== system mvdc_curvvel_tracking/CurvatureController/FeedForward/Curvature2Delta/InverseSteadyStateLinearModel/NeutralSteer ==
  CurvatureRequest_radpm : Inport
  Gain4 : Gain  Gain=l_front_m+l_rear_m
  SteeringAngle_rad : Outport
  wires:
  CurvatureRequest_radpm/1 -> Gain4/1
  Gain4/1 -> SteeringAngle_rad/1

== system mvdc_curvvel_tracking/CurvatureController/FeedForward/Curvature2Delta/InverseSteadyStateLinearModel/USCompensation_LinearModel ==
  VehicleVelocity_mps : Inport
  CurvatureRequest_radpm : Inport  Port=2
  Constant1 : Constant  Value=P_VDC_UndersteerGradient
  Constant4 : Constant  Value=P_VDC_UndersteerCompensationLowPassActive_b
  Product1 : Product  Inputs=3
  Product2 : Product
  Switch2 : Switch  Criteria=u2 > Threshold
  Transfer Fcn First Order : simulink/Discrete/Transfer Fcn First Order  PoleZ=exp(-tS/P_VDC_LowPassUSCT1)  ICPrevOutput=0.0  DoSatur=off
      settings: SourceProductName=Simulink
  USComp_SteeringAngle_rad : Outport
  wires:
  Constant1/1 -> Product1/3
  Product1/1 -> Product2/1
  Product2/1 -> Transfer Fcn First Order/1, Switch2/3
  Transfer Fcn First Order/1 -> Switch2/1
  Constant4/1 -> Switch2/2
  VehicleVelocity_mps/1 -> Product1/2, Product1/1
  CurvatureRequest_radpm/1 -> Product2/2
  Switch2/1 -> USComp_SteeringAngle_rad/1

== stateflow chart mvdc_curvvel_tracking/ControllerStateMachine/Chart ==
  state NormalOperation
    state FastControl
      entry:
      ControlState = TUMControlState.Fast;
      ActivateStandstill = false;
      LatFeedForward = true;
      LatFeedbackProportional = true;
      LatDisturbanceComp = true;
      LatActive = true;
      LongFeedForward = true;
      LongFeedbackProportional = true;
      LongDisturbanceComp = true;
      LongDisturbanceFF = true;
      LongActive = true;
    state SlowControl
      entry:
      ControlState = TUMControlState.Slow;
      ActivateStandstill = false;
      LatFeedForward = true;
      LatFeedbackProportional = true;
      LatDisturbanceComp = false;
      LatActive = true;
      LongFeedForward = false;
      LongFeedbackProportional = true;
      LongDisturbanceComp = false;
      LongDisturbanceFF = false;
      LongActive = true;
    FastControl -> SlowControl : [v_abs_mps < P_VDC_SlowControlSpeed_mps]
    SlowControl -> FastControl : [v_abs_mps > P_VDC_FullControlSpeed_mps]
  state EmergencyActive
    entry:
    ControlState = TUMControlState.Emergency;
    ActivateStandstill = false;
    LatFeedForward = true;
    LatFeedbackProportional = true;
    LatDisturbanceComp = true;
    LatActive = true;
    LongFeedForward = true;
    LongFeedbackProportional = false;
    LongDisturbanceComp = false;
    LongDisturbanceFF = false;
    LongActive = true;
  state BrakingControl
    entry:
    ControlState = TUMControlState.Brake;
    BrakeVelocity_mps = v_abs_mps;
    ActivateBrakeControl = true;
    during:
    BrakeVelocity_mps = BrakeVelocity_mps + tS*BrakeAcceleration_mps2;
  state RequestStandstill
    entry:
    ActivateStandstill = true;
  state DisableDrive
    entry: ParkBrakeActive = true;
  state StandstillControl
    entry:
    ControlState = TUMControlState.Standstill;
    ActivateStandstill = true;
    ActivateBrakeControl = false;
    LatFeedForward = false;
    LatFeedbackProportional = false;
    LatDisturbanceComp = false;
    LatActive = false;
    LongFeedForward = false;
    LongFeedbackProportional = false;
    LongDisturbanceComp = false;
    LongDisturbanceFF = false;
    LongActive = true;
    ParkBrakeActive = true;
  state DisableParkBrake
    entry: ParkBrakeActive = false;
  EmergencyActive -> BrakingControl : [~EnableDriving]
      | {BrakeAcceleration_mps2 = ...
      | P_VDC_EmergencyBrakeAcceleration_mps2;}
  NormalOperation -> BrakingControl [order 2] : [~EnableDriving]
      | {BrakeAcceleration_mps2 = ...
      | P_VDC_EmergencyBrakeAcceleration_mps2*0.5;}
  NormalOperation -> EmergencyActive [order 1] : [EmergencyActive]
  BrakingControl -> RequestStandstill : [v_abs_mps < P_VDC_EnterStandstillThreshhold_mps]
  RequestStandstill -> DisableDrive : after(0.5, sec)
  DisableParkBrake -> SlowControl : after(1, sec)
  DisableDrive -> StandstillControl : after(0.5, sec)
  StandstillControl -> DisableParkBrake : [EnableDriving]
  (default) -> StandstillControl
  data: v_abs_mps input; P_VDC_EnterStandstillThreshhold_mps parameter; P_VDC_SlowControlSpeed_mps parameter; P_VDC_FullControlSpeed_mps parameter; EnableDriving input boolean; LatFeedForward output boolean; LatFeedbackProportional output boolean; LatDisturbanceComp output boolean; LatActive output boolean; LongFeedForward output boolean; LongFeedbackProportional output boolean; LongDisturbanceComp output boolean; LongDisturbanceFF output boolean; LongActive output boolean; ActivateStandstill output boolean; ActivateBrakeControl output boolean; BrakeVelocity_mps output; BrakeAcceleration_mps2 output; P_VDC_EmergencyBrakeAcceleration_mps2 parameter; tS parameter; EmergencyActive input boolean; ControlState output Enum: TUMControlState; ParkBrakeActive output boolean
